simulink model "SporadicImpulse_Trajectory_Tests"  (R2019a)
settings: Solver=VariableStepAuto  StartTime=0.0  StopTime=40  RelTol=1e-3
InitFcn:
  | Sporadic_Impulse_3DOF_init
values from neighbouring files (symbols this model uses):
  g = 9.81    [Sporadic_Impulse_3DOF_init.m]    (also in Sporadic_Impulse_6DOF_init.m)
libraries: aerolibconvert2 x2, aerolibtransform2 x2, dspsrcs4 x1, aerolib3dof2 x1
settings Model: Creator=Devansh  LastModifiedBy=Devansh

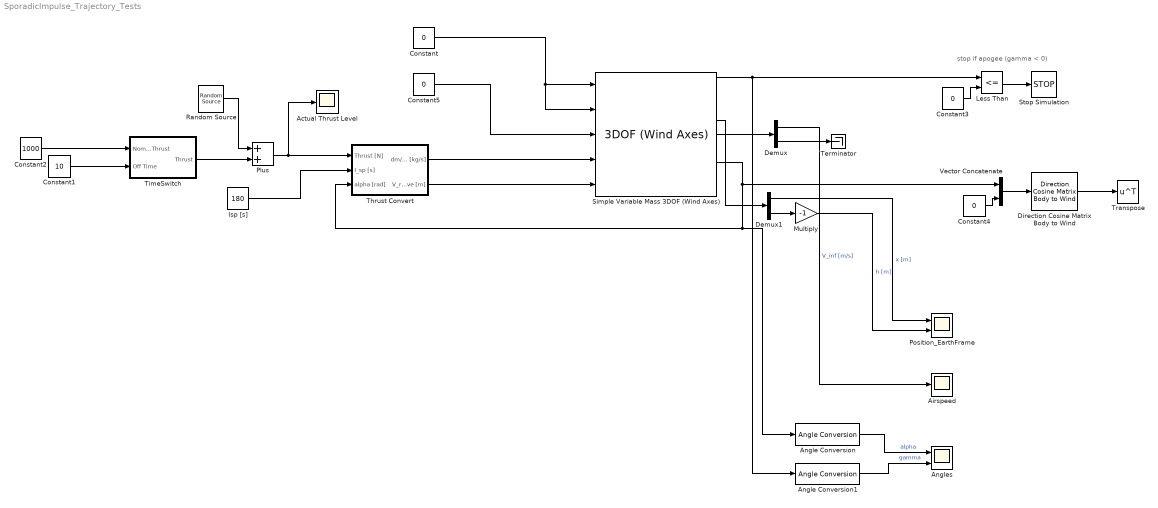
== system SporadicImpulse_Trajectory_Tests ==
  note: stop if apogee (gamma < 0)
  Actual Thrust Level : Scope
  Airspeed : Scope
  Angle Conversion : aerolibconvert2/Angle Conversion  IU=rad  OU=deg
  Angle Conversion1 : aerolibconvert2/Angle Conversion  IU=rad  OU=deg
  Angles : Scope  NumInputPorts=2
  Constant{,3..5} (4 alike) : Constant  Value=0
  Constant1 : Constant  Value=10
  Constant2 : Constant  Value=1000
  Demux : Demux  Outputs=2
  Demux1 : Demux  Outputs=2
  Direction Cosine Matrix Body to Wind : aerolibtransform2/Direction Cosine Matrix Body to Wind
      settings: SourceProductName=Aerospace Blockset  SourceProductBaseCode=AE
  Isp [s] : Constant  Value=180
  Less Than : RelationalOperator  Operator=<=  OutDataTypeStr=boolean  RndMeth=Simplest
  Multiply : Gain  Gain=-1
  Plus : Sum
  Position_EarthFrame : Scope  NumInputPorts=2
  Random Source : dspsrcs4/Random Source  SrcType=Gaussian  NormMethod=Ziggurat  CltLength=12  MinVal=0  MaxVal=1  MeanVal=0  VarVal=2500  RepMode=Not repeatable  rawSeed=1  IsInherit=off  SampMode=Discrete  SampTime=1  SampFrame=1  DataType=Double  OutComplex=Real  OutputFrames=off
  Simple Variable Mass 3DOF (Wind Axes) : aerolib3dof2/3DOF (Wind Axes)  units=Metric (MKS)  mtype=Simple Variable  V_ini=V_0  alpha_ini=alpha_0  gamma_ini=gamma_0  q_ini=0  pos_ini=[0 0]  mass=m_0  mass_e=m_dry  mass_f=m_0  Iyy=1.0  Iyy_e=I_dry  Iyy_f=I_0  g_in=Internal  g=g  vre_flag=on  abi_flag=on  V_statename=''  alpha_statename=''  gamma_statename=''  q_statename=''  pos_statename=''  mass_statename=''
      settings: SourceProductName=Aerospace Blockset  SourceProductBaseCode=AE
  Stop Simulation : Stop
  Terminator : Terminator
  Thrust Convert : Subsystem
  "TimeSwitch " : Subsystem
  Transpose : Math  Operator=transpose  SaturateOnIntegerOverflow=on
  Vector Concatenate : Concatenate
  wires:
  Constant/1 -> Simple Variable Mass 3DOF (Wind Axes)/2, Simple Variable Mass 3DOF (Wind Axes)/1
  Constant5/1 -> Simple Variable Mass 3DOF (Wind Axes)/3
  Simple Variable Mass 3DOF (Wind Axes)/7 -> Vector Concatenate/1, Thrust Convert/3(alpha [rad]), Angle Conversion/1
  Plus/1 -> Actual Thrust Level/1, Thrust Convert/1(Thrust [N])
  Isp [s]/1 -> Thrust Convert/2(I_sp [s])
  Thrust Convert/1(dm/dt [kg/s]) -> Simple Variable Mass 3DOF (Wind Axes)/4
  Thrust Convert/2(V_relative [m]) -> Simple Variable Mass 3DOF (Wind Axes)/5
  Simple Variable Mass 3DOF (Wind Axes)/5 -> Demux/1
  Demux/1 -> Airspeed/1  "V_inf [m/s]"
  Simple Variable Mass 3DOF (Wind Axes)/4 -> Demux1/1
  Demux1/2 -> Multiply/1
  Multiply/1 -> Position_EarthFrame/2  "h [m]"
  Demux1/1 -> Position_EarthFrame/1  "x [m]"
  Demux/2 -> Terminator/1
  Constant2/1 -> "TimeSwitch "/1(Nominal Thrust)
  Constant1/1 -> "TimeSwitch "/2(Off Time)
  Random Source/1 -> Plus/1
  "TimeSwitch "/1(Thrust) -> Plus/2
  Simple Variable Mass 3DOF (Wind Axes)/1 -> Angle Conversion1/1, Less Than/1
  Angle Conversion/1 -> Angles/1  "alpha"
  Angle Conversion1/1 -> Angles/2  "gamma"
  Constant3/1 -> Less Than/2
  Less Than/1 -> Stop Simulation/1
  Constant4/1 -> Vector Concatenate/2
  Vector Concatenate/1 -> Direction Cosine Matrix Body to Wind/1
  Direction Cosine Matrix Body to Wind/1 -> Transpose/1

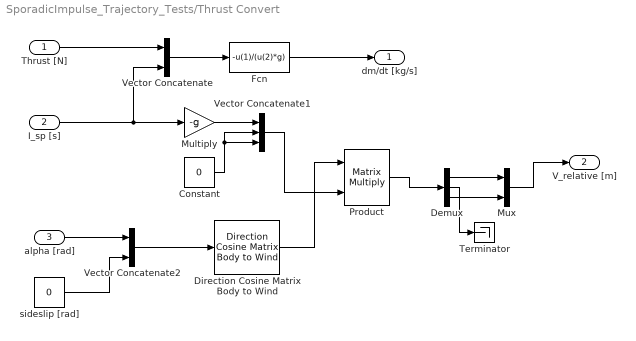
== system SporadicImpulse_Trajectory_Tests/Thrust Convert ==
  Thrust [N] : Inport
  I_sp [s] : Inport  Port=2
  alpha [rad] : Inport  Port=3
  Constant : Constant  Value=0
  Demux : Demux  Outputs=3
  Direction Cosine Matrix Body to Wind : aerolibtransform2/Direction Cosine Matrix Body to Wind
      settings: SourceProductName=Aerospace Blockset  SourceProductBaseCode=AE
  Fcn : Fcn  Expr=-u(1)/(u(2)*g)
  Multiply : Gain  Gain=-g
  Mux : Mux  Inputs=2
  Product : Product  Multiplication=Matrix(*)
  Terminator : Terminator
  Vector Concatenate : Concatenate
  Vector Concatenate1 : Concatenate  NumInputs=3
  Vector Concatenate2 : Concatenate
  sideslip [rad] : Constant  Value=0
  dm/dt [kg/s] : Outport
  V_relative [m] : Outport  Port=2
  wires:
  I_sp [s]/1 -> Multiply/1, Vector Concatenate/2
  Fcn/1 -> dm/dt [kg/s]/1
  Thrust [N]/1 -> Vector Concatenate/1
  Vector Concatenate/1 -> Fcn/1
  Constant/1 -> Vector Concatenate1/3, Vector Concatenate1/2
  Multiply/1 -> Vector Concatenate1/1
  alpha [rad]/1 -> Vector Concatenate2/1
  sideslip [rad]/1 -> Vector Concatenate2/2
  Vector Concatenate2/1 -> Direction Cosine Matrix Body to Wind/1
  Direction Cosine Matrix Body to Wind/1 -> Product/1
  Vector Concatenate1/1 -> Product/2
  Product/1 -> Demux/1
  Demux/1 -> Mux/1
  Mux/1 -> V_relative [m]/1
  Demux/3 -> Mux/2
  Demux/2 -> Terminator/1

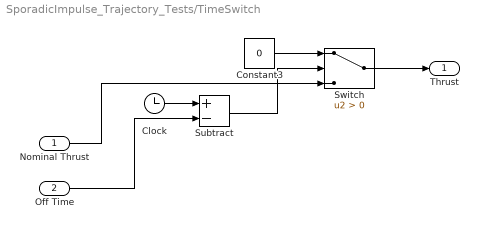
== system SporadicImpulse_Trajectory_Tests/TimeSwitch  ==
  Nominal Thrust : Inport
  Off Time : Inport  Port=2
  Clock : Clock
  Constant3 : Constant  Value=0
  Subtract : Sum  Inputs=+-
  Switch : Switch  Criteria=u2 > Threshold
  Thrust : Outport
  wires:
  Constant3/1 -> Switch/1
  Off Time/1 -> Subtract/2
  Nominal Thrust/1 -> Switch/3
  Clock/1 -> Subtract/1
  Switch/1 -> Thrust/1
  Subtract/1 -> Switch/2
